simulink model "sm_dcrank_aiming_mechanism_v1"  (R2021b)
settings: Solver=ode45  StartTime=0.0  StopTime=10.0  RelTol=1e-3  EnableMultiTasking=on
undefined symbols (not defined in the file or in its folder): sigbuilder_block, X, Y, Z
libraries: sm_lib x23, nesl_utility x4
Description:
  | Double Crank Aiming Mechanism
  | 
  | Aiming mechanism that points link A at a certain angle (beta). The mechanism is controlled by a PD controller that exerts a control torque at the joint Ri.
settings Model: FPTRunName=Active  Creator=The MathWorks, Inc.  LastModifiedBy=The MathWorks, Inc.
settings SolverCC: AlgebraicLoopSolver=TrustRegion
settings DataIOCC: LimitDataPoints=on  SaveFormat=Array  ReturnWorkspaceOutputs=off
settings OptimizationCC: OptimizeBlockIOStorage=off  BufferReuse=off  GlobalBufferReuse=off  ExpressionFolding=off  ExpressionDepthLimit=2147483647  LocalBlockOutputs=off  LifeSpan=inf  OptimizeDataStoreBuffers=off  BusAssignmentInplaceUpdate=off
settings DebuggingCC: UnderspecifiedInitializationDetection=Classic  MergeDetectMultiDrivingBlocksExec=none  FcnCallInpInsideContextMsg=warning  StateNameClashWarn=warning  SFUnexpectedBacktrackingDiag=warning  SFNoUnconditionalDefaultTransitionDiag=warning  SFExecutionAtInitializationDiag=none  SFMachineParentedDataDiag=warning  ArithmeticOperatorsInVariantConditions=warning
settings HardwareCC: ProdBitPerPointer=32  ProdBitPerSizeT=32  ProdBitPerPtrDiffT=32  ProdLargestAtomicFloat=None  ProdIntDivRoundTo=Undefined  ProdEndianess=Unspecified  ProdWordSize=32  ProdHWDeviceType=32-bit Generic
settings ModelReferenceCC: PropagateSignalLabelsOutOfModel=off
settings SFSimCC: SimUseLocalCustomCode=off  CustomCodeUndefinedFunction=UseInterfaceOnly
settings RTWCC: RTWUseLocalCustomCode=off
settings CodeAppCC: StateflowObjectComments=on
settings GRTTargetCC: TargetLangStandard=C89/C90 (ANSI)  CombineOutputUpdateFcns=off  GRTInterface=on
settings ConfigComp: CovMetricSettings=dw  CovSaveCumulativeToWorkspaceVar=on  CovSaveSingleToWorkspaceVar=on  CovExternalEMLEnable=off  CovSFcnEnable=off
settings SimscapeCC: SimscapeNormalizeSystem=off
settings ConfigurationSet: Description=SimMechanics 2G
settings DiagnosticsConfigSet: SimMechanicsUnconnectedFramePorts=none
settings ExplorerConfigSet: InternalSimMechanicsExplorerSettings="<ExplorerConfiguration><canonicalview>default</canonicalview><TilePanel><TileInfo><Tiles Columns=\"1\" Count=\"1\" Rows=\"1\"><Column Left=\"2\" Weight=\"1\"/><Column Left=\"460\"/><Row Top=\"2\" Weight=\"1\"/><Row Top=\"419\"/><Tile Height=\"1\" Width=\"1\" X=\"0\" Y=\"0\"/></Tiles></TileInfo><SceneInfo><SceneViewer><BGColor><R>0.60000002384185791</R><G>0.60000002384185791</G><B>0.60000002384185791</B></BGColor><Camera><Position><X>0.32766082882881165</X><Y>-0.9295329153538413</Y><Z>0.22762209177017212</Z></Position><Center><X>0.32766082882881165</X><Y>0</Y><Z>0.22762209177017212</Z></Center><Up><X>0</X><Y>-0</Y><Z>1</Z></Up><Left>-0.35608898699283603</Left><Right>0.35608898699283603</Right><Bottom>-0.26000320762395862</Bottom><Top>0.26000320762395862</Top></Camera></SceneViewer></SceneInfo></TilePanel></ExplorerConfiguration>"

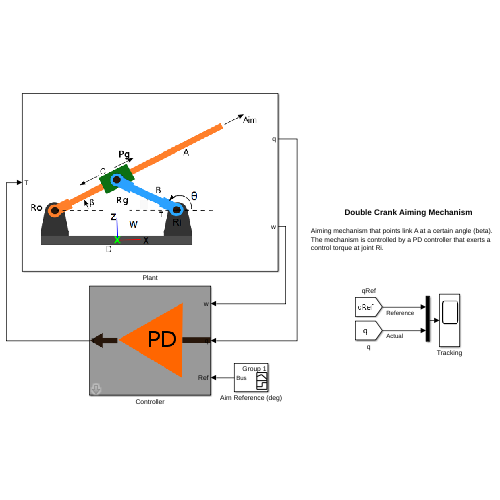
[thumbnail: Simulink's stored preview of the top-level diagram]
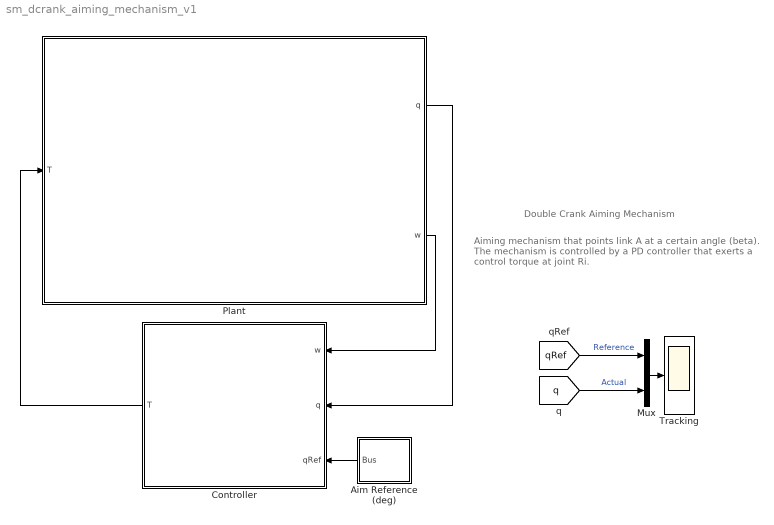
== system sm_dcrank_aiming_mechanism_v1 ==
  note: Double Crank Aiming Mechanism
  note: Aiming mechanism that points link A at a certain angle (beta).
      | The mechanism is controlled by a PD controller that exerts a
      | control torque at joint Ri.
  Aim Reference (deg) : Subsystem  Tag=STV Subsys  LoadFcn=sigbuilder_block('load');  StartFcn=sigbuilder_block('start');  StopFcn=sigbuilder_block('stop');  ClipboardFcn=sigbuilder_block('clipboard');  mask(Sigbuilder block){tuvar=[0:10]}
      mask help: Simulink:masks:SigbuilderBlock_MD
      mask init:
      | if ~strcmp(get_param(bdroot(gcbh),'SimulationStatus'),'stopped') tuvar = sigbuilder_block('maskInit'); end
      settings: CopyFcn=sigbuilder_block('copy');  DeleteFcn=sigbuilder_block('delete');  ModelCloseFcn=sigbuilder_block('modelClose');  PreSaveFcn=sigbuilder_block('preSave');  PauseFcn=sigbuilder_block('pause');  ContinueFcn=sigbuilder_block('continue');  NameChangeFcn=sigbuilder_block('namechange');  OpenFcn=sigbuilder_block('open',[437.6 199.2 550.4 400 ]);  CloseFcn=sigbuilder_block('close');
      mask Display: plot(0, 0, 100, 100,[2, 2, 32, 32, 2], [68, 8, 8, 68, 68],[32, 2], [38, 38], [32, 19, 2],[53, 60, 44], [32, 17, 17, 2],[16, 16, 31, 31]);txt = getActiveGroup(gcbh);text(2, 100, txt,'verticalAlignment', 'top');
  Controller : Subsystem  mask(PID Controller){Kp=500, Kd=50, Lb=30, Ld=40}
      mask prompts: Kp "Proportional Gain"; Kd "Derivative Gain"; Lb "Length of Link B (cm)"; Ld "Length of Link D (cm)"
      mask Display:
      | image('sm_dcrankaim_ctrl.png');
      | port_label('output',1,'T');
      | port_label('input',1,'w');
      | port_label('input',2,'q');
      | port_label('input',3,'Ref');
  Mux : Mux  Inputs=2
  Plant : Subsystem
      mask Display:
      | image('sm_aiming_mechanism.png');
      | port_label('input',1,'T');
      | port_label('output',1,'q');
      | port_label('output',2,'w');
  Tracking : Scope
  wires:
  Plant/2(w) -> Controller/1(w)
  Plant/1(q) -> Controller/2(q)
  Controller/1(T) -> Plant/1(T)
  Mux/1 -> Tracking/1
  [q] -> Mux/2  "Actual"
  [qRef] -> Mux/1  "Reference"
  Aim Reference (deg)/1(Bus) -> Controller/3(qRef)

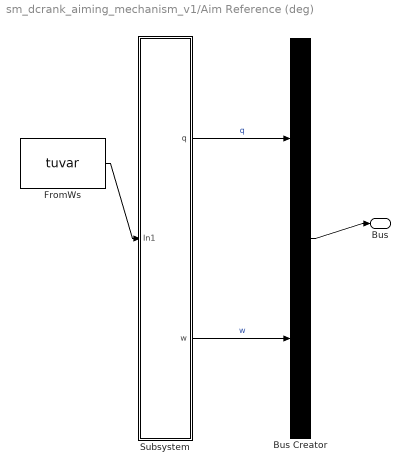
== system sm_dcrank_aiming_mechanism_v1/Aim Reference (deg) ==
  Bus Creator : BusCreator  Tag=Bus Creator  Inputs=2
  FromWs : FromWorkspace  Tag=STV FromWs  VariableName=tuvar
      SigBuilderData=|
      | common.afterFinalStr = 'Extrapolate'
      | common.sampleTime = 0
      | dataSet.timeRange = [0 10]
      | dataSet.name = 'Group 1'
      | sbobj.Groups.Name = 'Group 1'
      | sbobj.Groups.Signals(1).Name = 'q'
      | sbobj.Groups.Signals(1).XData = [0 2 2 4 4 6 6 8 8 10]
      | sbobj.Groups.Signals(1).YData = [10 10 45 45 5 5 35 35 20 20]
      | sbobj.Groups.Signals(2).Name = 'w'
      | sbobj.Groups.Signals(2).XData = [0 10]
      | sbobj.Groups.Signals(2).YData = [0 0]
  Subsystem : Subsystem
  Bus : Outport  VectorParamsAs1DForOutWhenUnconnected=off
  wires:
  FromWs/1 -> Subsystem/1(In1)
  Subsystem/1(q) -> Bus Creator/1  "q"
  Subsystem/2(w) -> Bus Creator/2  "w"
  Bus Creator/1 -> Bus/1

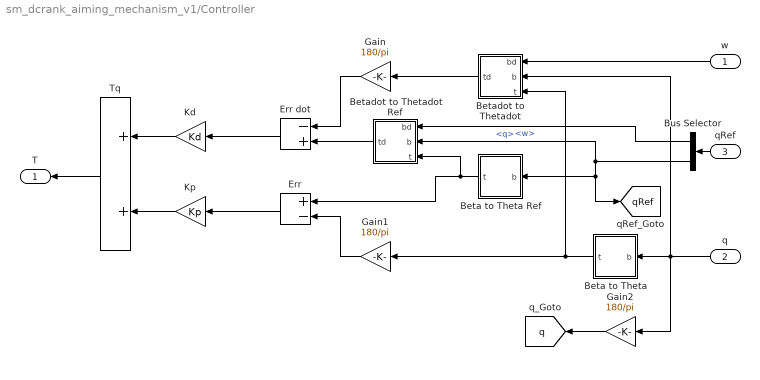
== system sm_dcrank_aiming_mechanism_v1/Controller ==
  w : Inport
  q : Inport  Port=2
  qRef : Inport  Port=3
  Beta to Theta : Subsystem
  Beta to Theta Ref : Subsystem
  Betadot to Thetadot : Subsystem
  Betadot to Thetadot Ref : Subsystem
  Bus Selector : BusSelector  OutputSignals=w,q
  Err : Sum  Inputs=+-
  Err dot : Sum  Inputs=-+
  Gain : Gain  Gain=180/pi
  Gain1 : Gain  Gain=180/pi
  Gain2 : Gain  Gain=180/pi
  Kd : Gain  Gain=Kd
  Kp : Gain  Gain=Kp
  Tq : Sum
  T : Outport  VectorParamsAs1DForOutWhenUnconnected=off
  tag scope: q=global, qRef=global
  wires:
  Gain/1 -> Err dot/1
  Gain1/1 -> Err/2
  Err dot/1 -> Kd/1
  Err/1 -> Kp/1
  Tq/1 -> T/1
  Kp/1 -> Tq/2
  q/1 -> Beta to Theta/1(b), Betadot to Thetadot/2(b), Gain2/1
  Beta to Theta/1(t) -> Gain1/1, Betadot to Thetadot/3(t)
  Beta to Theta Ref/1(t) -> Err/1, Betadot to Thetadot Ref/3(t)
  w/1 -> Betadot to Thetadot/1(bd)
  Betadot to Thetadot/1(td) -> Gain/1
  Gain2/1 -> [q]
  Kd/1 -> Tq/1
  qRef/1 -> Bus Selector/1
  Betadot to Thetadot Ref/1(td) -> Err dot/2
  Bus Selector/2 -> Beta to Theta Ref/1(b), [qRef], Betadot to Thetadot Ref/2(b)  "<q>"
  Bus Selector/1 -> Betadot to Thetadot Ref/1(bd)  "<w>"

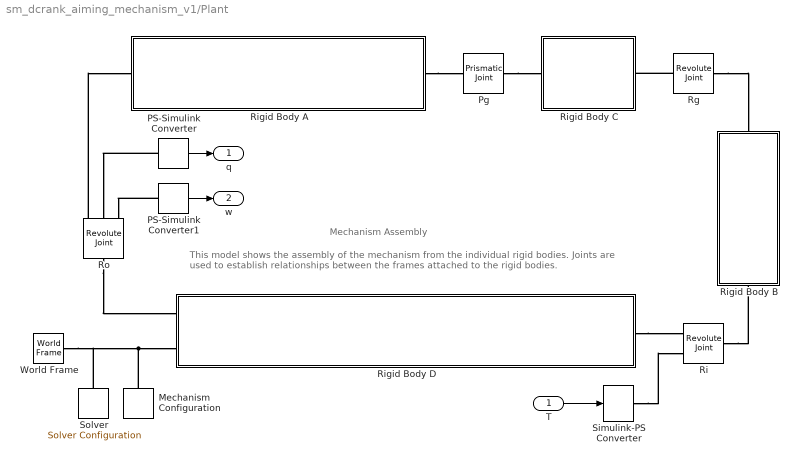
== system sm_dcrank_aiming_mechanism_v1/Plant ==
  note: Mechanism Assembly
  note: This model shows the assembly of the mechanism from the individual rigid bodies. Joints
      | are used to establish relationships between the frames attached to the rigid bodies.
  T : Inport
  Mechanism Configuration : sm_lib/Utilities/Mechanism Configuration  UniformGravity=Constant  GravityVector=[0 0 -9.81]  GravityUnits=m/s^2  LinearizationDelta=0.001  JointModeTransitionNonlinearIterations=2
  PS-Simulink Converter : nesl_utility/PS-Simulink Converter  PhysicalDomain=network_engine_domain  SubClassName=ps_output  LeftPortType=input  RightPortType=output  PseudoPeriodic=off  Frequencies=[]  Unit=rad  AffineConversion=off
      settings: SourceProductBaseCode=PW,SS
  PS-Simulink Converter1 : nesl_utility/PS-Simulink Converter  PhysicalDomain=network_engine_domain  SubClassName=ps_output  LeftPortType=input  RightPortType=output  PseudoPeriodic=off  Frequencies=[]  Unit=rad/s  AffineConversion=off
      settings: SourceProductBaseCode=PW,SS
  Pg : sm_lib/Joints/Prismatic Joint  JointMode=Normal  SenseConstraintForce=off  SenseConstraintForceX=off  SenseConstraintForceY=off  SenseConstraintForceZ=off  SenseConstraintTorque=off  SenseConstraintTorqueX=off  SenseConstraintTorqueY=off  SenseConstraintTorqueZ=off  SenseTotalForce=off  SenseTotalForceX=off  SenseTotalForceY=off  SenseTotalForceZ=off  SenseTotalTorque=off  SenseTotalTorqueX=off  SenseTotalTorqueY=off  SenseTotalTorqueZ=off  CompositeWrenchDir=FollowerOnBase  CompositeWrenchFrame=BaseFrame  EquilibriumPosition=0  EquilibriumPositionUnits=m  SpringStiffness=0  SpringStiffnessUnits=N/m  DampingCoefficient=0  DampingCoefficientUnits=N/(m/s)  TorqueActuationMode=NoTorque  MotionActuationMode=ComputedMotion  SensePosition=off  SenseVelocity=off  SenseAcceleration=off  SenseTorqueForce=off  SenseLowerLimitTorqueForce=off  SenseUpperLimitTorqueForce=off  LowerLimitSpecify=off  LowerLimitBound=-1  LowerLimitBoundUnits=m  LowerLimitStiffness=1e6  LowerLimitStiffnessUnits=N/m  LowerLimitDamping=1e3  LowerLimitDampingUnits=N/(m/s)  LowerLimitTransitionRegionWidth=1e-4  LowerLimitTransitionRegionWidthUnits=m  UpperLimitSpecify=off  UpperLimitBound=1  UpperLimitBoundUnits=m  UpperLimitStiffness=1e6  UpperLimitStiffnessUnits=N/m  UpperLimitDamping=1e3  UpperLimitDampingUnits=N/(m/s)  UpperLimitTransitionRegionWidth=1e-4  UpperLimitTransitionRegionWidthUnits=m  PositionTargetSpecify=off  PositionTargetPriority=High  PositionTargetValue=0  PositionTargetValueUnits=m  VelocityTargetSpecify=off  VelocityTargetPriority=High  VelocityTargetValue=0  VelocityTargetValueUnits=m/s
  Rg : sm_lib/Joints/Revolute Joint  JointMode=Normal  SenseConstraintForce=off  SenseConstraintForceX=off  SenseConstraintForceY=off  SenseConstraintForceZ=off  SenseConstraintTorque=off  SenseConstraintTorqueX=off  SenseConstraintTorqueY=off  SenseConstraintTorqueZ=off  SenseTotalForce=off  SenseTotalForceX=off  SenseTotalForceY=off  SenseTotalForceZ=off  SenseTotalTorque=off  SenseTotalTorqueX=off  SenseTotalTorqueY=off  SenseTotalTorqueZ=off  CompositeWrenchDir=FollowerOnBase  CompositeWrenchFrame=BaseFrame  EquilibriumPosition=0  EquilibriumPositionUnits=rad  SpringStiffness=0  SpringStiffnessUnits=N*m/rad  DampingCoefficient=0  DampingCoefficientUnits=N*m/(rad/s)  TorqueActuationMode=NoTorque  MotionActuationMode=ComputedMotion  SensePosition=off  SenseVelocity=off  SenseAcceleration=off  SenseTorqueForce=off  SenseLowerLimitTorqueForce=off  SenseUpperLimitTorqueForce=off  LowerLimitSpecify=off  LowerLimitBound=-90  LowerLimitBoundUnits=deg  LowerLimitStiffness=1e4  LowerLimitStiffnessUnits=N*m/deg  LowerLimitDamping=10  LowerLimitDampingUnits=N*m/(deg/s)  LowerLimitTransitionRegionWidth=0.1  LowerLimitTransitionRegionWidthUnits=deg  UpperLimitSpecify=off  UpperLimitBound=90  UpperLimitBoundUnits=deg  UpperLimitStiffness=1e4  UpperLimitStiffnessUnits=N*m/deg  UpperLimitDamping=10  UpperLimitDampingUnits=N*m/(deg/s)  UpperLimitTransitionRegionWidth=0.1  UpperLimitTransitionRegionWidthUnits=deg  PositionTargetSpecify=off  PositionTargetPriority=High  PositionTargetValue=0  PositionTargetValueUnits=rad  VelocityTargetSpecify=off  VelocityTargetPriority=High  VelocityTargetValue=0  VelocityTargetValueUnits=rad/s
  Ri : sm_lib/Joints/Revolute Joint  JointMode=Normal  SenseConstraintForce=off  SenseConstraintForceX=off  SenseConstraintForceY=off  SenseConstraintForceZ=off  SenseConstraintTorque=off  SenseConstraintTorqueX=off  SenseConstraintTorqueY=off  SenseConstraintTorqueZ=off  SenseTotalForce=off  SenseTotalForceX=off  SenseTotalForceY=off  SenseTotalForceZ=off  SenseTotalTorque=off  SenseTotalTorqueX=off  SenseTotalTorqueY=off  SenseTotalTorqueZ=off  CompositeWrenchDir=FollowerOnBase  CompositeWrenchFrame=BaseFrame  EquilibriumPosition=0  EquilibriumPositionUnits=rad  SpringStiffness=0  SpringStiffnessUnits=N*m/rad  DampingCoefficient=0  DampingCoefficientUnits=N*m/(rad/s)  TorqueActuationMode=InputTorque  MotionActuationMode=ComputedMotion  SensePosition=off  SenseVelocity=off  SenseAcceleration=off  SenseTorqueForce=off  SenseLowerLimitTorqueForce=off  SenseUpperLimitTorqueForce=off  LowerLimitSpecify=off  LowerLimitBound=-90  LowerLimitBoundUnits=deg  LowerLimitStiffness=1e4  LowerLimitStiffnessUnits=N*m/deg  LowerLimitDamping=10  LowerLimitDampingUnits=N*m/(deg/s)  LowerLimitTransitionRegionWidth=0.1  LowerLimitTransitionRegionWidthUnits=deg  UpperLimitSpecify=off  UpperLimitBound=90  UpperLimitBoundUnits=deg  UpperLimitStiffness=1e4  UpperLimitStiffnessUnits=N*m/deg  UpperLimitDamping=10  UpperLimitDampingUnits=N*m/(deg/s)  UpperLimitTransitionRegionWidth=0.1  UpperLimitTransitionRegionWidthUnits=deg  PositionTargetSpecify=on  PositionTargetPriority=Low  PositionTargetValue=150  PositionTargetValueUnits=deg  VelocityTargetSpecify=off  VelocityTargetPriority=High  VelocityTargetValue=0  VelocityTargetValueUnits=rad/s
  Rigid Body A : Subsystem  mask(First Approximation of Rigid Body A){L=80, R=2, rho=2700}
      mask prompts: L "Length of Link (cm)"; R "Radius of Link (cm)"; rho "Density of Link (kg/m^3)"
      mask help:
      | This subsystem represents a first approximation of the rigid body A.
      | Right click on the block and select "Look Under Mask" to view the components that make up the rigid body.
      mask Display:
      | image('sm_dcrankaim_approx_body_A_act.png')
      | port_label('LConn',1,'Fad')
      | port_label('RConn',1,'Fac')
  Rigid Body B : Subsystem  mask(First Approximation of Rigid Body B){L=30, R=2, rho=2700}
      mask prompts: L "Length of Link (cm)"; R "Radius of Link (cm)"; rho "Density of Link (kg/m^3)"
      mask help:
      | This subsystem represents a first approximation of the rigid body B.
      | Right click on the block and select "Look Under Mask" to view the components that make up the rigid body.
      mask Display:
      | image('sm_dcrankaim_approx_body_B_act.png')
      | port_label('LConn',1,'Fbd')
      | port_label('RConn',1,'Fbc')
  Rigid Body C : Subsystem  mask(First Approximation of Rigid Body C){L=10, B=8, H=8, rho=2700}
      mask prompts: L "Length of Link (cm)"; B "Breadth of Link (cm)"; H "Height of Link (cm)"; rho "Density of Link (kg/m^3)"
      mask help:
      | This subsystem represents a first approximation of the rigid body C.
      | Right click on the block and select "Look Under Mask" to view the components that make up the rigid body.
      mask Display:
      | image('sm_dcrankaim_approx_body_C_act.png')
      | port_label('LConn',1,'Fca')
      | port_label('RConn',1,'Fcb')
  Rigid Body D : Subsystem  mask(First Approximation of Rigid Body D){L=40, R=2, rho=2700}
      mask prompts: L "Length of Link (cm)"; R "Radius of Link (cm)"; rho "Density of Link (kg/m^3)"
      mask help:
      | This subsystem represents a first approximation of the rigid body D.
      | Right click on the block and select "Look Under Mask" to view the components that make up the rigid body.
      mask Display:
      | image('sm_dcrankaim_approx_body_D_act.png')
      | port_label('LConn',1,'Fda')
      | port_label('LConn',2,'Fdw')
      | port_label('RConn',1,'Fdb')
  Ro : sm_lib/Joints/Revolute Joint  JointMode=Normal  SenseConstraintForce=off  SenseConstraintForceX=off  SenseConstraintForceY=off  SenseConstraintForceZ=off  SenseConstraintTorque=off  SenseConstraintTorqueX=off  SenseConstraintTorqueY=off  SenseConstraintTorqueZ=off  SenseTotalForce=off  SenseTotalForceX=off  SenseTotalForceY=off  SenseTotalForceZ=off  SenseTotalTorque=off  SenseTotalTorqueX=off  SenseTotalTorqueY=off  SenseTotalTorqueZ=off  CompositeWrenchDir=FollowerOnBase  CompositeWrenchFrame=BaseFrame  EquilibriumPosition=0  EquilibriumPositionUnits=rad  SpringStiffness=0  SpringStiffnessUnits=N*m/rad  DampingCoefficient=0  DampingCoefficientUnits=N*m/(rad/s)  TorqueActuationMode=NoTorque  MotionActuationMode=ComputedMotion  SensePosition=on  SenseVelocity=on  SenseAcceleration=off  SenseTorqueForce=off  SenseLowerLimitTorqueForce=off  SenseUpperLimitTorqueForce=off  LowerLimitSpecify=off  LowerLimitBound=-90  LowerLimitBoundUnits=deg  LowerLimitStiffness=1e4  LowerLimitStiffnessUnits=N*m/deg  LowerLimitDamping=10  LowerLimitDampingUnits=N*m/(deg/s)  LowerLimitTransitionRegionWidth=0.1  LowerLimitTransitionRegionWidthUnits=deg  UpperLimitSpecify=off  UpperLimitBound=90  UpperLimitBoundUnits=deg  UpperLimitStiffness=1e4  UpperLimitStiffnessUnits=N*m/deg  UpperLimitDamping=10  UpperLimitDampingUnits=N*m/(deg/s)  UpperLimitTransitionRegionWidth=0.1  UpperLimitTransitionRegionWidthUnits=deg  PositionTargetSpecify=on  PositionTargetPriority=High  PositionTargetValue=35  PositionTargetValueUnits=deg  VelocityTargetSpecify=off  VelocityTargetPriority=High  VelocityTargetValue=0  VelocityTargetValueUnits=rad/s
  Simulink-PS Converter : nesl_utility/Simulink-PS Converter  PhysicalDomain=network_engine_domain  SubClassName=ps_input  LeftPortType=input  RightPortType=output  PseudoPeriodic=off  Frequencies=[]  NoiseDistribution=none  NoiseParameters=[]  Unit=N*m  AffineConversion=off  FilteringAndDerivatives=zero  SimscapeFilterOrder=1  InputFilterTimeConstant=.001  UdotUserProvided=1
      settings: SourceProductBaseCode=PW,SS
  Solver : nesl_utility/Solver Configuration  PhysicalDomain=network_engine_domain  SubClassName=solver  LeftPortType=input  RightPortType=generic  Tones=[]  Harmonics=[]  SimulateNoise=off  Profile=off  UseLocalSampling=off  EnableSwitchedLinearOptims=on  FrequencyDomain=off  UseCCode=off  RelTol=0.001  AbsTol=1e-06  MinStep=1e-09  ToWorkspace=off  RevertToSquareIcSolve=off  NumHomotopyIterations=100  PhasorMode=off  PhasorModeNumHarmonics=1  DoDC=off  ResidualTolerance=1e-9  UseLocalSolver=off  LocalSolverChoice=NE_BACKWARD_EULER_ADVANCER  LocalSolverSampleTime=.001  DoFixedCost=off  MaxNonlinIter=3  MaxModeIter=2  ComputeImpulses=off  ImpulseIterations=2  LinearAlgebra=Sparse  EquationFormulation=NE_TIME_EF  DelaysMemoryBudget=1024  AutomaticFiltering=on  FilteringTimeConstant=0.001  PartitionStorageMethod=AS_NEEDED  PartitionMemoryBudget=1024  PartitionMethod=FAST
      settings: SourceProductBaseCode=PW,SS
  World Frame : sm_lib/Frames and Transforms/World Frame
  q : Outport  VectorParamsAs1DForOutWhenUnconnected=off
  w : Outport  Port=2  VectorParamsAs1DForOutWhenUnconnected=off
  wires:
  PS-Simulink Converter/1 -> q/1
  T/1 -> Simulink-PS Converter/1
  PS-Simulink Converter1/1 -> w/1
  connections:
  Mechanism Configuration/RConn1 -- World Frame/RConn1 -- Solver/RConn1 -- Rigid Body D/LConn2
  PS-Simulink Converter/LConn1 -- Ro/RConn2
  Rigid Body A/RConn1 -- Pg/LConn1
  Pg/RConn1 -- Rigid Body C/LConn1
  Ro/RConn1 -- Rigid Body A/LConn1
  Ro/LConn1 -- Rigid Body D/LConn1
  PS-Simulink Converter1/LConn1 -- Ro/RConn3
  Rigid Body D/RConn1 -- Ri/LConn1
  Ri/RConn1 -- Rigid Body B/LConn1
  Simulink-PS Converter/RConn1 -- Ri/LConn2
  Rg/LConn1 -- Rigid Body B/RConn1
  Rg/RConn1 -- Rigid Body C/RConn1

== system sm_dcrank_aiming_mechanism_v1/Aim Reference (deg)/Subsystem ==
  In1 : Inport
  Demux : Demux  Tag=STV Demux  Outputs=2
      settings: DisplayOption=none
  q : Outport  Tag=STV Outport  VectorParamsAs1DForOutWhenUnconnected=off
  w : Outport  Tag=STV Outport  Port=2  VectorParamsAs1DForOutWhenUnconnected=off
  wires:
  Demux/1 -> q/1
  Demux/2 -> w/1
  In1/1 -> Demux/1

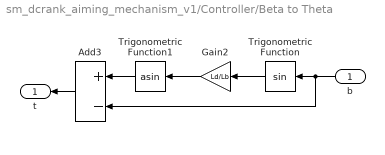
== system sm_dcrank_aiming_mechanism_v1/Controller/Beta to Theta ==
  b : Inport
  Add3 : Sum  Inputs=+-
  Gain2 : Gain  Gain=Ld/Lb
  Trigonometric Function : Trigonometry
  Trigonometric Function1 : Trigonometry  Operator=asin
  t : Outport  VectorParamsAs1DForOutWhenUnconnected=off
  wires:
  b/1 -> Trigonometric Function/1, Add3/2
  Trigonometric Function/1 -> Gain2/1
  Gain2/1 -> Trigonometric Function1/1
  Trigonometric Function1/1 -> Add3/1
  Add3/1 -> t/1

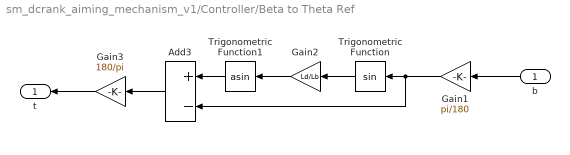
== system sm_dcrank_aiming_mechanism_v1/Controller/Beta to Theta Ref ==
  b : Inport
  Add3 : Sum  Inputs=+-
  Gain1 : Gain  Gain=pi/180
  Gain2 : Gain  Gain=Ld/Lb
  Gain3 : Gain  Gain=180/pi
  Trigonometric Function : Trigonometry
  Trigonometric Function1 : Trigonometry  Operator=asin
  t : Outport  VectorParamsAs1DForOutWhenUnconnected=off
  wires:
  Add3/1 -> Gain3/1
  Trigonometric Function1/1 -> Add3/1
  Gain2/1 -> Trigonometric Function1/1
  Trigonometric Function/1 -> Gain2/1
  b/1 -> Gain1/1
  Gain1/1 -> Add3/2, Trigonometric Function/1
  Gain3/1 -> t/1

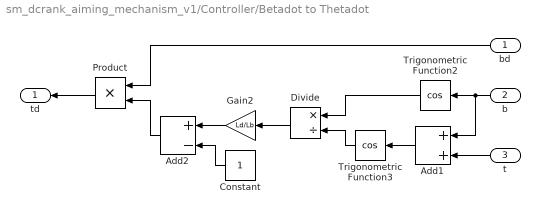
== system sm_dcrank_aiming_mechanism_v1/Controller/Betadot to Thetadot ==
  bd : Inport
  b : Inport  Port=2
  t : Inport  Port=3
  Add1 : Sum
  Add2 : Sum  Inputs=+-
  Constant : Constant
  Divide : Product  Inputs=*/
  Gain2 : Gain  Gain=Ld/Lb
  Product : Product  RndMeth=Zero
  Trigonometric Function2 : Trigonometry  Operator=cos
  Trigonometric Function3 : Trigonometry  Operator=cos
  td : Outport  VectorParamsAs1DForOutWhenUnconnected=off
  wires:
  Product/1 -> td/1
  b/1 -> Trigonometric Function2/1, Add1/1
  t/1 -> Add1/2
  Add1/1 -> Trigonometric Function3/1
  Trigonometric Function3/1 -> Divide/2
  Trigonometric Function2/1 -> Divide/1
  Divide/1 -> Gain2/1
  Gain2/1 -> Add2/1
  Constant/1 -> Add2/2
  bd/1 -> Product/1
  Add2/1 -> Product/2

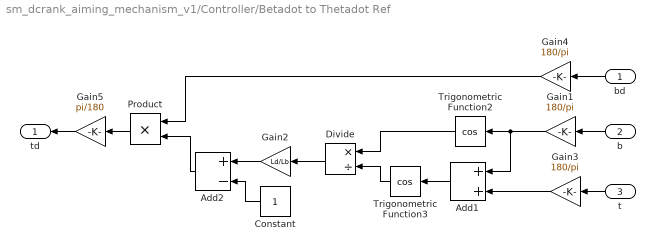
== system sm_dcrank_aiming_mechanism_v1/Controller/Betadot to Thetadot Ref ==
  bd : Inport
  b : Inport  Port=2
  t : Inport  Port=3
  Add1 : Sum
  Add2 : Sum  Inputs=+-
  Constant : Constant
  Divide : Product  Inputs=*/
  Gain1 : Gain  Gain=180/pi
  Gain2 : Gain  Gain=Ld/Lb
  Gain3 : Gain  Gain=180/pi
  Gain4 : Gain  Gain=180/pi
  Gain5 : Gain  Gain=pi/180
  Product : Product  RndMeth=Zero
  Trigonometric Function2 : Trigonometry  Operator=cos
  Trigonometric Function3 : Trigonometry  Operator=cos
  td : Outport  VectorParamsAs1DForOutWhenUnconnected=off
  wires:
  Add2/1 -> Product/2
  bd/1 -> Gain4/1
  Constant/1 -> Add2/2
  Gain2/1 -> Add2/1
  Divide/1 -> Gain2/1
  Trigonometric Function2/1 -> Divide/1
  Trigonometric Function3/1 -> Divide/2
  Add1/1 -> Trigonometric Function3/1
  t/1 -> Gain3/1
  b/1 -> Gain1/1
  Product/1 -> Gain5/1
  Gain1/1 -> Add1/1, Trigonometric Function2/1
  Gain3/1 -> Add1/2
  Gain4/1 -> Product/1
  Gain5/1 -> td/1

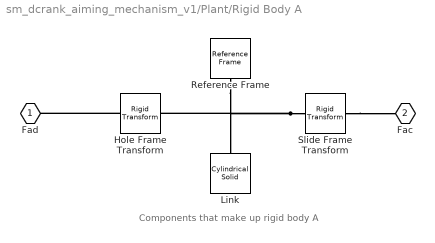
== system sm_dcrank_aiming_mechanism_v1/Plant/Rigid Body A ==
  note: Components that make up rigid body A
  Hole Frame Transform : sm_lib/Frames and Transforms/Rigid Transform  TranslationMethod=StandardAxis  TranslationStandardOffset=L/2  TranslationLengthUnit=cm  TranslationStandardAxis=-Z  TranslationCartesianOffset=[0 0 0]  TranslationROffset=0  TranslationROffsetUnits=m  TranslationZOffset=0  TranslationZOffsetUnits=m  TranslationThetaOffset=0  TranslationThetaOffsetUnits=deg  RotationMethod=AlignedAxes  RotationAngleUnits=deg  RotationStandardAxis=+Z  RotationAngle=0  RotationArbitraryAxis=[0 0 1]  FollAlignAxisA=+Z  BaseAlignAxisA=-Y  FollAlignAxisB=+X  BaseAlignAxisB=+Z  RotationSequenceAxes=FollowerAxes  RotationSequence=XYX  RotationSequenceAngles=[0 0 0]  RotationSequenceAnglesUnits=deg  RotationMatrix=[1 0 0; 0 1 0; 0 0 1]
  Link : sm_lib/Body Elements/Cylindrical Solid  GraphicAmbientColor=[0.5 0.5 0.5]  BasedOnType=Density  CenterOfMass=[0 0 0]  CenterOfMassUnits=m  GraphicDiffuseColor=[1.0 0.4 0.0]  CylinderLength=L  CylinderLengthUnits=cm  CylinderRadius=R  CylinderRadiusUnits=cm  Density=rho  DensityUnits=kg/m^3  DoExposeReferenceFrame=on  GraphicEmissiveColor=[0.1 0.1 0.1]  ExportEntireGeometry=off  SerializedFrames=<Frames/>  MarkerShape=Sphere  MarkerSize=1  GraphicType=FromGeometry  InertiaType=CalculateFromGeometry  Mass=1  MassUnits=kg  MomentsOfInertia=[1 1 1]  MomentsOfInertiaUnits=kg*m^2  GraphicOpacity=1  ProductsOfInertia=[0 0 0]  ProductsOfInertiaUnits=kg*m^2  GraphicShininess=24.0  GraphicSpecularColor=[0.2 0.2 0.2]  GraphicVisPropType=SimpleVisualProperties
  Reference Frame : sm_lib/Frames and Transforms/Reference Frame
  Slide Frame Transform : sm_lib/Frames and Transforms/Rigid Transform  TranslationMethod=None  TranslationStandardOffset=0  TranslationLengthUnit=cm  TranslationStandardAxis=+Z  TranslationCartesianOffset=[0 0 0]  TranslationROffset=0  TranslationROffsetUnits=m  TranslationZOffset=0  TranslationZOffsetUnits=m  TranslationThetaOffset=0  TranslationThetaOffsetUnits=deg  RotationMethod=AlignedAxes  RotationAngleUnits=deg  RotationStandardAxis=+Z  RotationAngle=0  RotationArbitraryAxis=[0 0 1]  FollAlignAxisA=+Y  BaseAlignAxisA=-X  FollAlignAxisB=+X  BaseAlignAxisB=+Y  RotationSequenceAxes=FollowerAxes  RotationSequence=XYX  RotationSequenceAngles=[0 0 0]  RotationSequenceAnglesUnits=deg  RotationMatrix=[1 0 0; 0 1 0; 0 0 1]
  Fad : PMIOPort  Side=Left
  Fac : PMIOPort  Port=2  Side=Right
  connections:
  Slide Frame Transform/LConn1 -- Hole Frame Transform/LConn1 -- Link/RConn1 -- Reference Frame/RConn1
  Hole Frame Transform/RConn1 -- Fad/RConn1
  Slide Frame Transform/RConn1 -- Fac/RConn1

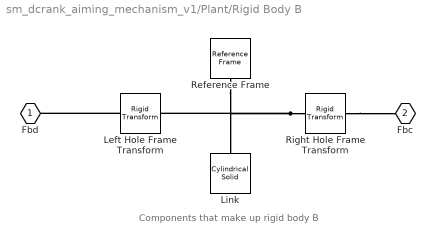
== system sm_dcrank_aiming_mechanism_v1/Plant/Rigid Body B ==
  note: Components that make up rigid body B
  Left Hole Frame Transform : sm_lib/Frames and Transforms/Rigid Transform  TranslationMethod=StandardAxis  TranslationStandardOffset=L/2  TranslationLengthUnit=cm  TranslationStandardAxis=-Z  TranslationCartesianOffset=[0 0 0]  TranslationROffset=0  TranslationROffsetUnits=m  TranslationZOffset=0  TranslationZOffsetUnits=m  TranslationThetaOffset=0  TranslationThetaOffsetUnits=deg  RotationMethod=AlignedAxes  RotationAngleUnits=deg  RotationStandardAxis=+Z  RotationAngle=0  RotationArbitraryAxis=[0 0 1]  FollAlignAxisA=+Z  BaseAlignAxisA=-Y  FollAlignAxisB=+X  BaseAlignAxisB=+Z  RotationSequenceAxes=FollowerAxes  RotationSequence=XYX  RotationSequenceAngles=[0 0 0]  RotationSequenceAnglesUnits=deg  RotationMatrix=[1 0 0; 0 1 0; 0 0 1]
  Link : sm_lib/Body Elements/Cylindrical Solid  GraphicAmbientColor=[0.5 0.5 0.5]  BasedOnType=Density  CenterOfMass=[0 0 0]  CenterOfMassUnits=m  GraphicDiffuseColor=[0.0 0.6 0.8]  CylinderLength=L  CylinderLengthUnits=cm  CylinderRadius=R  CylinderRadiusUnits=cm  Density=rho  DensityUnits=kg/m^3  DoExposeReferenceFrame=on  GraphicEmissiveColor=[0.1 0.1 0.1]  ExportEntireGeometry=off  SerializedFrames=<Frames/>  MarkerShape=Sphere  MarkerSize=1  GraphicType=FromGeometry  InertiaType=CalculateFromGeometry  Mass=1  MassUnits=kg  MomentsOfInertia=[1 1 1]  MomentsOfInertiaUnits=kg*m^2  GraphicOpacity=1  ProductsOfInertia=[0 0 0]  ProductsOfInertiaUnits=kg*m^2  GraphicShininess=24.0  GraphicSpecularColor=[0.2 0.2 0.2]  GraphicVisPropType=SimpleVisualProperties
  Reference Frame : sm_lib/Frames and Transforms/Reference Frame
  Right Hole Frame Transform : sm_lib/Frames and Transforms/Rigid Transform  TranslationMethod=StandardAxis  TranslationStandardOffset=L/2  TranslationLengthUnit=cm  TranslationStandardAxis=+Z  TranslationCartesianOffset=[0 0 0]  TranslationROffset=0  TranslationROffsetUnits=m  TranslationZOffset=0  TranslationZOffsetUnits=m  TranslationThetaOffset=0  TranslationThetaOffsetUnits=deg  RotationMethod=AlignedAxes  RotationAngleUnits=deg  RotationStandardAxis=+Z  RotationAngle=0  RotationArbitraryAxis=[0 0 1]  FollAlignAxisA=+Z  BaseAlignAxisA=-Y  FollAlignAxisB=+X  BaseAlignAxisB=+Z  RotationSequenceAxes=FollowerAxes  RotationSequence=XYX  RotationSequenceAngles=[0 0 0]  RotationSequenceAnglesUnits=deg  RotationMatrix=[1 0 0; 0 1 0; 0 0 1]
  Fbd : PMIOPort  Side=Left
  Fbc : PMIOPort  Port=2  Side=Right
  connections:
  Right Hole Frame Transform/LConn1 -- Left Hole Frame Transform/LConn1 -- Link/RConn1 -- Reference Frame/RConn1
  Left Hole Frame Transform/RConn1 -- Fbd/RConn1
  Right Hole Frame Transform/RConn1 -- Fbc/RConn1

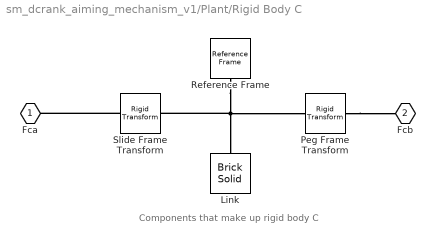
== system sm_dcrank_aiming_mechanism_v1/Plant/Rigid Body C ==
  note: Components that make up rigid body C
  Link : sm_lib/Body Elements/Brick Solid  GraphicAmbientColor=[0.5 0.5 0.5]  BasedOnType=Density  BrickDimensions=[L B H]  BrickDimensionUnits=cm  CenterOfMass=[0 0 0]  CenterOfMassUnits=m  GraphicDiffuseColor=[0.0 0.6 0.0]  Density=rho  DensityUnits=kg/m^3  DoExposeReferenceFrame=on  GraphicEmissiveColor=[0.1 0.1 0.1]  ExportEntireGeometry=off  SerializedFrames=<Frames/>  MarkerShape=Sphere  MarkerSize=1  GraphicType=FromGeometry  InertiaType=CalculateFromGeometry  Mass=1  MassUnits=kg  MomentsOfInertia=[1 1 1]  MomentsOfInertiaUnits=kg*m^2  GraphicOpacity=0.7  ProductsOfInertia=[0 0 0]  ProductsOfInertiaUnits=kg*m^2  GraphicShininess=24.0  GraphicSpecularColor=[0.2 0.2 0.2]  GraphicVisPropType=SimpleVisualProperties
  Peg Frame Transform : sm_lib/Frames and Transforms/Rigid Transform  TranslationMethod=None  TranslationStandardOffset=0  TranslationLengthUnit=cm  TranslationStandardAxis=+Z  TranslationCartesianOffset=[0 0 0]  TranslationROffset=0  TranslationROffsetUnits=m  TranslationZOffset=0  TranslationZOffsetUnits=m  TranslationThetaOffset=0  TranslationThetaOffsetUnits=deg  RotationMethod=AlignedAxes  RotationAngleUnits=deg  RotationStandardAxis=+Z  RotationAngle=0  RotationArbitraryAxis=[0 0 1]  FollAlignAxisA=+Z  BaseAlignAxisA=-Y  FollAlignAxisB=+Y  BaseAlignAxisB=+Z  RotationSequenceAxes=FollowerAxes  RotationSequence=XYX  RotationSequenceAngles=[0 0 0]  RotationSequenceAnglesUnits=deg  RotationMatrix=[1 0 0; 0 1 0; 0 0 1]
  Reference Frame : sm_lib/Frames and Transforms/Reference Frame
  Slide Frame Transform : sm_lib/Frames and Transforms/Rigid Transform  TranslationMethod=None  TranslationStandardOffset=0  TranslationLengthUnit=cm  TranslationStandardAxis=-Z  TranslationCartesianOffset=[0 0 0]  TranslationROffset=0  TranslationROffsetUnits=m  TranslationZOffset=0  TranslationZOffsetUnits=m  TranslationThetaOffset=0  TranslationThetaOffsetUnits=deg  RotationMethod=AlignedAxes  RotationAngleUnits=deg  RotationStandardAxis=+Z  RotationAngle=0  RotationArbitraryAxis=[0 0 1]  FollAlignAxisA=+Z  BaseAlignAxisA=+X  FollAlignAxisB=+Y  BaseAlignAxisB=+Z  RotationSequenceAxes=FollowerAxes  RotationSequence=XYX  RotationSequenceAngles=[0 0 0]  RotationSequenceAnglesUnits=deg  RotationMatrix=[1 0 0; 0 1 0; 0 0 1]
  Fca : PMIOPort  Side=Left
  Fcb : PMIOPort  Port=2  Side=Right
  connections:
  Peg Frame Transform/RConn1 -- Fcb/RConn1
  Slide Frame Transform/RConn1 -- Fca/RConn1
  Reference Frame/RConn1 -- Link/RConn1 -- Slide Frame Transform/LConn1 -- Peg Frame Transform/LConn1

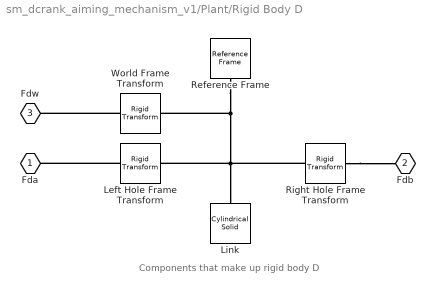
== system sm_dcrank_aiming_mechanism_v1/Plant/Rigid Body D ==
  note: Components that make up rigid body D
  Left Hole Frame Transform : sm_lib/Frames and Transforms/Rigid Transform  TranslationMethod=StandardAxis  TranslationStandardOffset=L/2  TranslationLengthUnit=cm  TranslationStandardAxis=-Z  TranslationCartesianOffset=[0 0 0]  TranslationROffset=0  TranslationROffsetUnits=m  TranslationZOffset=0  TranslationZOffsetUnits=m  TranslationThetaOffset=0  TranslationThetaOffsetUnits=deg  RotationMethod=AlignedAxes  RotationAngleUnits=deg  RotationStandardAxis=+Z  RotationAngle=0  RotationArbitraryAxis=[0 0 1]  FollAlignAxisA=+Z  BaseAlignAxisA=-Y  FollAlignAxisB=+X  BaseAlignAxisB=+Z  RotationSequenceAxes=FollowerAxes  RotationSequence=XYX  RotationSequenceAngles=[0 0 0]  RotationSequenceAnglesUnits=deg  RotationMatrix=[1 0 0; 0 1 0; 0 0 1]
  Link : sm_lib/Body Elements/Cylindrical Solid  GraphicAmbientColor=[0.5 0.5 0.5]  BasedOnType=Density  CenterOfMass=[0 0 0]  CenterOfMassUnits=m  GraphicDiffuseColor=[0.4 0.4 0.4]  CylinderLength=L  CylinderLengthUnits=cm  CylinderRadius=R  CylinderRadiusUnits=cm  Density=rho  DensityUnits=kg/m^3  DoExposeReferenceFrame=on  GraphicEmissiveColor=[0.1 0.1 0.1]  ExportEntireGeometry=off  SerializedFrames=<Frames/>  MarkerShape=Sphere  MarkerSize=1  GraphicType=FromGeometry  InertiaType=CalculateFromGeometry  Mass=1  MassUnits=kg  MomentsOfInertia=[1 1 1]  MomentsOfInertiaUnits=kg*m^2  GraphicOpacity=1  ProductsOfInertia=[0 0 0]  ProductsOfInertiaUnits=kg*m^2  GraphicShininess=24.0  GraphicSpecularColor=[0.2 0.2 0.2]  GraphicVisPropType=SimpleVisualProperties
  Reference Frame : sm_lib/Frames and Transforms/Reference Frame
  Right Hole Frame Transform : sm_lib/Frames and Transforms/Rigid Transform  TranslationMethod=StandardAxis  TranslationStandardOffset=L/2  TranslationLengthUnit=cm  TranslationStandardAxis=+Z  TranslationCartesianOffset=[0 0 0]  TranslationROffset=0  TranslationROffsetUnits=m  TranslationZOffset=0  TranslationZOffsetUnits=m  TranslationThetaOffset=0  TranslationThetaOffsetUnits=deg  RotationMethod=AlignedAxes  RotationAngleUnits=deg  RotationStandardAxis=+Z  RotationAngle=0  RotationArbitraryAxis=[0 0 1]  FollAlignAxisA=+Z  BaseAlignAxisA=-Y  FollAlignAxisB=+X  BaseAlignAxisB=+Z  RotationSequenceAxes=FollowerAxes  RotationSequence=XYX  RotationSequenceAngles=[0 0 0]  RotationSequenceAnglesUnits=deg  RotationMatrix=[1 0 0; 0 1 0; 0 0 1]
  World Frame Transform : sm_lib/Frames and Transforms/Rigid Transform  TranslationMethod=StandardAxis  TranslationStandardOffset=L/2  TranslationLengthUnit=cm  TranslationStandardAxis=-Z  TranslationCartesianOffset=[0 0 0]  TranslationROffset=0  TranslationROffsetUnits=m  TranslationZOffset=0  TranslationZOffsetUnits=m  TranslationThetaOffset=0  TranslationThetaOffsetUnits=deg  RotationMethod=AlignedAxes  RotationAngleUnits=deg  RotationStandardAxis=+Z  RotationAngle=0  RotationArbitraryAxis=[0 0 1]  FollAlignAxisA=+X  BaseAlignAxisA=+Z  FollAlignAxisB=+Z  BaseAlignAxisB=-X  RotationSequenceAxes=FollowerAxes  RotationSequence=XYX  RotationSequenceAngles=[0 0 0]  RotationSequenceAnglesUnits=deg  RotationMatrix=[1 0 0; 0 1 0; 0 0 1]
  Fda : PMIOPort  Side=Left
  Fdb : PMIOPort  Port=2  Side=Right
  Fdw : PMIOPort  Port=3  Side=Left
  connections:
  Right Hole Frame Transform/RConn1 -- Fdb/RConn1
  Left Hole Frame Transform/RConn1 -- Fda/RConn1
  Reference Frame/RConn1 -- Link/RConn1 -- Left Hole Frame Transform/LConn1 -- Right Hole Frame Transform/LConn1 -- World Frame Transform/LConn1
  World Frame Transform/RConn1 -- Fdw/RConn1
